simulink model "DUC"  (R2024b)
settings: Solver=VariableStepAuto  StartTime=0.0  StopTime=0.01  RelTol=1e-3
values from neighbouring files (symbols this model uses):
  compFilt = design(compSpec,'SystemObject',true)    [main.m]
  fs_base = 48e3    (= 48000)    [main.m]
  hbFilt = design(hbSpec,'SystemObject',true)    [main.m]
  lowpassFilt = design(lowpassSpec,'SystemObject',true)    [main.m]
  N4_cycle = 16    [main.m]
  outputframe = 1    [main.m]
  upsample_L = 128    [main.m]
libraries: dsphdlfiltering2 x8, dspsigops x2, dsphdlsigops2 x1, dspsrcs4 x1
settings Model: Creator=31651  LastModifiedBy=31651
settings OptimizationCC: BlockReduction=off  ConditionallyExecuteInputs=off
settings RTWCC: GPUComputeCapability=3.5

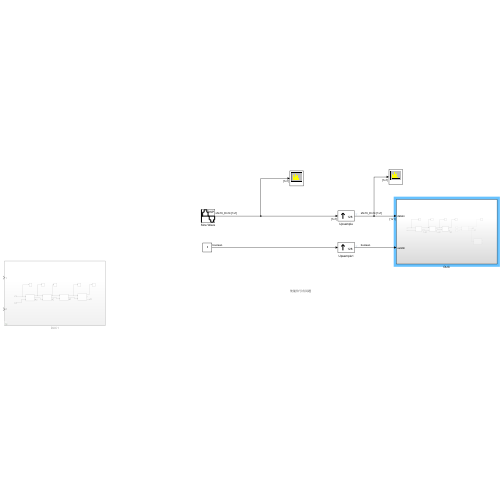
[thumbnail: Simulink's stored preview of the top-level diagram]
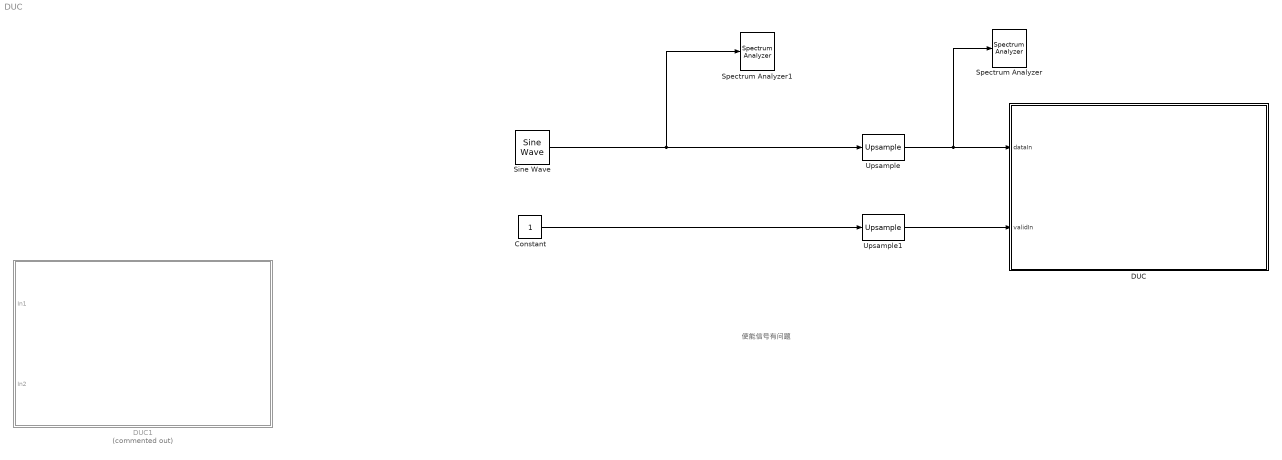
== system DUC ==
  note: 使能信号有问题
  Constant : Constant  OutDataTypeStr=boolean  SampleTime=1/fs_base
  DUC : Subsystem
  DUC1 : Subsystem  Commented=on
  Sine Wave : dspsrcs4/Sine Wave  Amplitude=0.49  Frequency=1000  Phase=0  SampleMode=Discrete  OutComplex=Real  CompMethod=Table lookup  TableSize=Speed  SampleTime=1/fs_base  SamplesPerFrame=1  ResetState=Restart at time zero  OutputFrames=off  dataType=Fixed-point  wordLen=16  udDataType=sfix(16)  fracBitsMode=User-defined  numFracBits=14  OutDataTypeStr=fixdt(1,16,14)  LastOutDataTypeStr=fixdt(1,16,14)
  Spectrum Analyzer : SpectrumAnalyzer  WindowPosition=[281.000000,455.000000,800.000000,500.000000,]  Visible=on  ScopeFrameLocation=window  Span=1536000  StartFrequency=-768000  StopFrequency=768000  YLimits=[-74.80002538,-15.17224138]
  Spectrum Analyzer1 : SpectrumAnalyzer  WindowPosition=[937.000000,87.000000,800.000000,500.000000,]  Visible=on  ScopeFrameLocation=window  Span=48000  StartFrequency=-24000  StopFrequency=24000  YLimits=[-67.06844200304198,41.7822128823489]
  Upsample : dspsigops/Upsample  FactorSource=Dialog parameter  N=ceil(upsample_L/outputframe)  Nmax=16  phase=0  RateOptions=Allow multirate processing  ic=0  mode=Unused parameter value
      settings: LibrarySourceBlock=dsphdlsupportsigops/Upsample
  Upsample1 : dspsigops/Upsample  FactorSource=Dialog parameter  N=ceil(upsample_L/outputframe)  Nmax=16  phase=0  RateOptions=Allow multirate processing  ic=0  mode=Unused parameter value
      settings: LibrarySourceBlock=dsphdlsupportsigops/Upsample
  wires:
  Constant/1 -> Upsample1/1
  Upsample/1 -> Spectrum Analyzer/1, DUC/1(dataIn)
  Upsample1/1 -> DUC/2(validIn)
  Sine Wave/1 -> Spectrum Analyzer1/1, Upsample/1

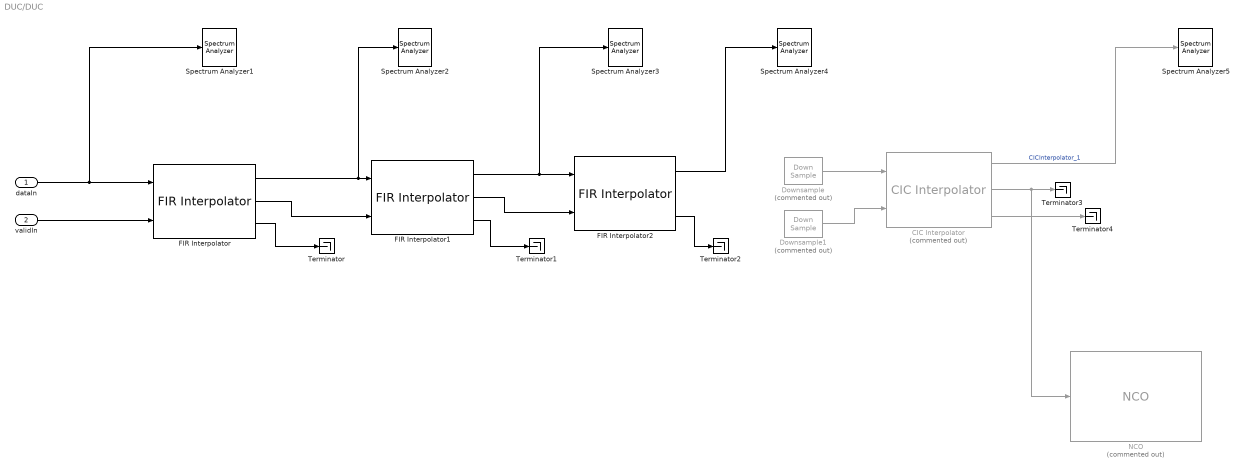
== system DUC/DUC ==
  dataIn : Inport
  validIn : Inport  Port=2
  CIC Interpolator : dsphdlfiltering2/CIC Interpolator  Commented=on  InterpolationSource=Property  InterpolationFactor=16  MaxInterpolationFactor=2  DifferentialDelay=1  NumSections=2  NumCycles=ceil(upsample_L/(outputframe*8))  GainCorrection=off  SimulateUsing=Code generation  OutputDataType=Minimum section word lengths  OutputWordLength=14  ResetInputPort=off  HDLGlobalReset=off
  Downsample : DownSample  Commented=on  N=N4_cycle  RateOptions=Allow multirate processing
  Downsample1 : DownSample  Commented=on  N=N4_cycle  RateOptions=Allow multirate processing
  FIR Interpolator : dsphdlfiltering2/FIR Interpolator  Numerator=lowpassFilt.Numerator  FilterStructure=Direct form systolic  InterpolationFactor=2  NumCycles=1  OptimizeSymmCoeff=off  SimulateUsing=Code generation  roundingMode=Floor  overflowMode=off  CoefficientsDataTypeStr=Inherit: Same word length as input  OutputDataTypeStr=fixdt(1,18,14)  ResetInputPort=off  HDLGlobalReset=off
  FIR Interpolator1 : dsphdlfiltering2/FIR Interpolator  Numerator=hbFilt.Numerator  FilterStructure=Direct form systolic  InterpolationFactor=2  NumCycles=1  OptimizeSymmCoeff=off  SimulateUsing=Code generation  roundingMode=Floor  overflowMode=off  CoefficientsDataTypeStr=Inherit: Same word length as input  OutputDataTypeStr=fixdt(1,18,14)  ResetInputPort=off  HDLGlobalReset=off
  FIR Interpolator2 : dsphdlfiltering2/FIR Interpolator  Numerator=compFilt.Numerator  FilterStructure=Direct form systolic  InterpolationFactor=2  NumCycles=1  OptimizeSymmCoeff=off  SimulateUsing=Code generation  roundingMode=Floor  overflowMode=off  CoefficientsDataTypeStr=Inherit: Same word length as input  OutputDataTypeStr=fixdt(1,18,14)  ResetInputPort=off  HDLGlobalReset=off
  NCO : dsphdlsigops2/NCO  Commented=on  PhaseIncrementSource=Property  PhaseIncrement=phInc  PhaseOffsetSource=Property  PhaseOffset=0  DitherSource=Property  NumDitherBits=ditherBits  SamplesPerFrame=outputframe  LUTCompress=off  ResetAction=off  Waveform=Sine  PhasePort=off  SimulateUsing=Code generation  AccumulatorWL=Nnco  PhaseQuantization=on  NumQuantizerAccumulatorBits=Q  OutputDataType=Binary point scaling  OutputWL=16  OutputFL=14
      settings: LibrarySourceBlock=dsphdlsrcs2/NCO
  Spectrum Analyzer1 : SpectrumAnalyzer  WindowPosition=[307.000000,645.000000,800.000000,500.000000,]  ScopeFrameLocation=window  Span=1536000  StartFrequency=-768000  StopFrequency=768000  YLimits=[-74.80002538,-15.17224138]
  Spectrum Analyzer2 : SpectrumAnalyzer  WindowPosition=[1309.000000,588.000000,800.000000,500.000000,]  ScopeFrameLocation=window  Span=1536000  StartFrequency=-768000  StopFrequency=768000  YLimits=[-125.84114105,-9.56376457]
  Spectrum Analyzer3 : SpectrumAnalyzer  WindowPosition=[998.000000,449.000000,800.000000,500.000000,]  ScopeFrameLocation=window  Span=1536000  StartFrequency=-768000  StopFrequency=768000  YLimits=[-130.13183393,-9.75110776]
  Spectrum Analyzer4 : SpectrumAnalyzer  WindowPosition=[687.000000,402.000000,800.000000,500.000000,]  ScopeFrameLocation=window  Span=1536000  StartFrequency=-768000  StopFrequency=768000  YLimits=[-67.83664152,-16.25429049]
  Spectrum Analyzer5 : SpectrumAnalyzer  WindowPosition=[996.000000,381.000000,800.000000,500.000000,]  ScopeFrameLocation=window  Span=6144000  StartFrequency=-3072000  StopFrequency=3072000  YLimits=[-3603.44492261,-2802.67938425]
  Terminator{,1..4} (5 alike) : Terminator
  wires:
  CIC Interpolator/3 -> Terminator4/1
  CIC Interpolator/2 -> NCO/1, Terminator3/1
  FIR Interpolator1/1 -> Spectrum Analyzer3/1, FIR Interpolator2/1
  FIR Interpolator2/1 -> Spectrum Analyzer4/1
  CIC Interpolator/1 -> Spectrum Analyzer5/1  "CICInterpolator_1"
  FIR Interpolator1/2 -> FIR Interpolator2/2
  dataIn/1 -> FIR Interpolator/1, Spectrum Analyzer1/1
  FIR Interpolator2/3 -> Terminator2/1
  FIR Interpolator1/3 -> Terminator1/1
  FIR Interpolator/3 -> Terminator/1
  validIn/1 -> FIR Interpolator/2
  FIR Interpolator/1 -> Spectrum Analyzer2/1, FIR Interpolator1/1
  FIR Interpolator/2 -> FIR Interpolator1/2
  Downsample/1 -> CIC Interpolator/1
  Downsample1/1 -> CIC Interpolator/2

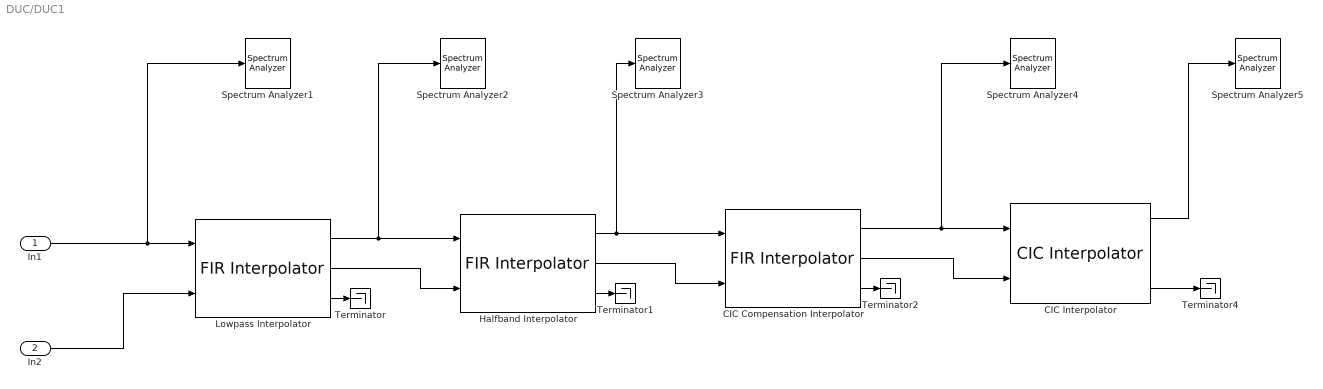
== system DUC/DUC1 ==
  In1 : Inport
  In2 : Inport  Port=2
  CIC Compensation Interpolator : dsphdlfiltering2/FIR Interpolator  Numerator=compFilt.Numerator  FilterStructure=Direct form systolic  InterpolationFactor=2  NumCycles=2  OptimizeSymmCoeff=off  SimulateUsing=Code generation  roundingMode=Floor  overflowMode=off  CoefficientsDataTypeStr=Inherit: Same word length as input  OutputDataTypeStr=fixdt(1,18,14)  ResetInputPort=off  HDLGlobalReset=off
  CIC Interpolator : dsphdlfiltering2/CIC Interpolator  InterpolationSource=Property  InterpolationFactor=16  MaxInterpolationFactor=2  DifferentialDelay=1  NumSections=4  NumCycles=1  GainCorrection=off  SimulateUsing=Code generation  OutputDataType=Minimum section word lengths  OutputWordLength=14  ResetInputPort=off  HDLGlobalReset=on
  Halfband Interpolator : dsphdlfiltering2/FIR Interpolator  Numerator=hbFilt.Numerator  FilterStructure=Direct form systolic  InterpolationFactor=2  NumCycles=4  OptimizeSymmCoeff=off  SimulateUsing=Code generation  roundingMode=Floor  overflowMode=off  CoefficientsDataTypeStr=Inherit: Same word length as input  OutputDataTypeStr=fixdt(1,18,14)  ResetInputPort=off  HDLGlobalReset=off
  Lowpass Interpolator : dsphdlfiltering2/FIR Interpolator  Numerator=lowpassFilt.Numerator  FilterStructure=Direct form systolic  InterpolationFactor=2  NumCycles=8  OptimizeSymmCoeff=off  SimulateUsing=Code generation  roundingMode=Floor  overflowMode=off  CoefficientsDataTypeStr=Inherit: Same word length as input  OutputDataTypeStr=fixdt(1,18,14)  ResetInputPort=off  HDLGlobalReset=off
  Spectrum Analyzer1 : SpectrumAnalyzer  WindowPosition=[880.000000,470.000000,800.000000,500.000000,]  ScopeFrameLocation=window  Span=384000  StartFrequency=-192000  StopFrequency=192000  YLimits=[-11.70247649,-4.58344478]
  Spectrum Analyzer2 : SpectrumAnalyzer  WindowPosition=[880.000000,470.000000,800.000000,500.000000,]  ScopeFrameLocation=window  Span=384000  StartFrequency=-192000  StopFrequency=192000  YLimits=[-95.85824329,11.61236288]
  Spectrum Analyzer3 : SpectrumAnalyzer  WindowPosition=[880.000000,470.000000,800.000000,500.000000,]  ScopeFrameLocation=window  Span=384000  StartFrequency=-192000  StopFrequency=192000  YLimits=[-116.23716208,20.65446958]
  Spectrum Analyzer4 : SpectrumAnalyzer  WindowPosition=[822.000000,315.000000,800.000000,500.000000,]  ScopeFrameLocation=window  Span=384000  StartFrequency=-192000  StopFrequency=192000  YLimits=[-111.54026712,26.95931223]
  Spectrum Analyzer5 : SpectrumAnalyzer  WindowPosition=[1271.000000,440.000000,800.000000,500.000000,]  ScopeFrameLocation=window  Span=6144000  StartFrequency=-3072000  StopFrequency=3072000  YLimits=[-14.69010096,108.0201507]
  Terminator{,1..2,4} (4 alike) : Terminator
  wires:
  CIC Interpolator/3 -> Terminator4/1
  Lowpass Interpolator/2 -> Halfband Interpolator/2
  Halfband Interpolator/1 -> Spectrum Analyzer3/1, CIC Compensation Interpolator/1
  CIC Compensation Interpolator/1 -> Spectrum Analyzer4/1, CIC Interpolator/1
  CIC Compensation Interpolator/2 -> CIC Interpolator/2
  Lowpass Interpolator/1 -> Spectrum Analyzer2/1, Halfband Interpolator/1
  CIC Interpolator/1 -> Spectrum Analyzer5/1
  Halfband Interpolator/2 -> CIC Compensation Interpolator/2
  In1/1 -> Spectrum Analyzer1/1, Lowpass Interpolator/1
  CIC Compensation Interpolator/3 -> Terminator2/1
  Halfband Interpolator/3 -> Terminator1/1
  Lowpass Interpolator/3 -> Terminator/1
  In2/1 -> Lowpass Interpolator/2
